simulink model "nucleo_g431re_ihm07m1"  (R2024a)
settings: Solver=FixedStepDiscrete  StartTime=0.0  StopTime=10  FixedStep=Ts  RelTol=1e-3  EnableMultiTasking=on
model workspace (MAT data in the model file):
  encoderResolution = 2000
  hallOffset = '0.5'
  indexOffset = 850
  polePairs = '4'
values from neighbouring files (symbols this model uses):
  motorParam =     [matlab.mat]
  PWM_Counter_Period = round(CPU_frequency/PWM_frequency/2)    [mcb_stm32_param_est_InitFunc.m]
  Ts = 1/PWM_frequency    (= 5e-05)    [mcb_stm32_param_est_InitFunc.m]    (also in stm32_pmsm_foc_data.m)
undefined symbols (not defined in the file or in its folder): DiscIntNeverNeededParam, inverter, NumBits1, NumBits2, Slope1, Slope2
libraries: mcbcontrolslib x24, simulink x15, stm32f4xxblockslib x4, stm32g4xxblockslib x3, slpidlib x2, stm32blockslib x2, svdutilitieslib x1
(part 2 of 3)

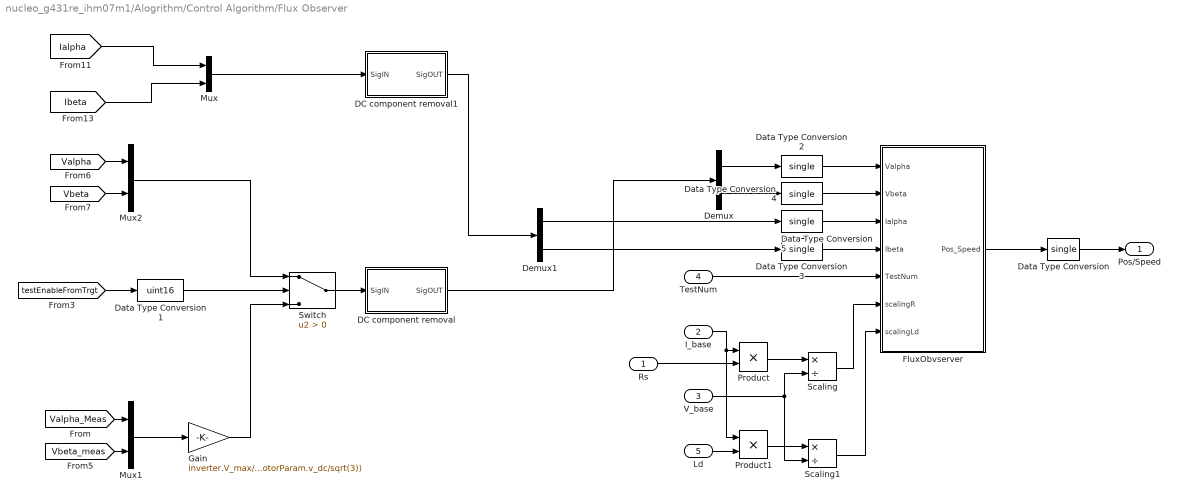
== system nucleo_g431re_ihm07m1/Alogrithm/Control Algorithm/Flux Observer ==
  Rs : Inport
  I_base : Inport  Port=2
  V_base : Inport  Port=3
  TestNum : Inport  Port=4
  Ld : Inport  Port=5
  DC component removal : Subsystem
  DC component removal1 : Subsystem
  Data Type Conversion{,2..5} (5 alike) : DataTypeConversion  OutDataTypeStr=single  RndMeth=Simplest  SaturateOnIntegerOverflow=off
  Data Type Conversion1 : DataTypeConversion  OutDataTypeStr=uint16  RndMeth=Simplest  SaturateOnIntegerOverflow=off
  Demux : Demux  Outputs=2
  Demux1 : Demux  Outputs=2
  FluxObvserver : Subsystem
  Gain : Gain  Gain=inverter.V_max/(motorParam.v_dc/sqrt(3))  RndMeth=Simplest  OutDataTypeStr=Inherit: Same as input
  Mux : Mux  Inputs=2
  Mux1 : Mux  Inputs=2
  Mux2 : Mux  Inputs=2
  Product : Product
  Product1 : Product
  Scaling : Product  Inputs=*/
  Scaling1 : Product  Inputs=*/
  Switch : Switch  Criteria=u2 > Threshold  SaturateOnIntegerOverflow=off  InputSameDT=off
  Pos/Speed : Outport  VectorParamsAs1DForOutWhenUnconnected=off
  wires:
  Data Type Conversion/1 -> Pos/Speed/1
  I_base/1 -> Product1/1, Product/1
  Rs/1 -> Product/2
  Product/1 -> Scaling/1
  [Ibeta] -> Mux/2
  [Ialpha] -> Mux/1
  Demux/2 -> Data Type Conversion4/1
  Demux/1 -> Data Type Conversion2/1
  FluxObvserver/1(Pos_Speed) -> Data Type Conversion/1
  Data Type Conversion2/1 -> FluxObvserver/1(Valpha)
  Data Type Conversion4/1 -> FluxObvserver/2(Vbeta)
  TestNum/1 -> FluxObvserver/5(TestNum)
  Scaling/1 -> FluxObvserver/6(scalingR)
  [Vbeta_meas] -> Mux1/2
  Mux1/1 -> Gain/1
  [Valpha_Meas] -> Mux1/1
  Gain/1 -> Switch/3
  V_base/1 -> Scaling/2, Scaling1/2
  Product1/1 -> Scaling1/1
  Ld/1 -> Product1/2
  Scaling1/1 -> FluxObvserver/7(scalingLd)
  Data Type Conversion1/1 -> Switch/2
  [Valpha] -> Mux2/1
  [Vbeta] -> Mux2/2
  Mux2/1 -> Switch/1
  [testEnableFromTrgt] -> Data Type Conversion1/1
  Data Type Conversion5/1 -> FluxObvserver/3(Ialpha)
  Data Type Conversion3/1 -> FluxObvserver/4(Ibeta)
  Switch/1 -> DC component removal/1(SigIN)
  DC component removal/1(SigOUT) -> Demux/1
  DC component removal1/1(SigOUT) -> Demux1/1
  Demux1/2 -> Data Type Conversion3/1
  Mux/1 -> DC component removal1/1(SigIN)
  Demux1/1 -> Data Type Conversion5/1

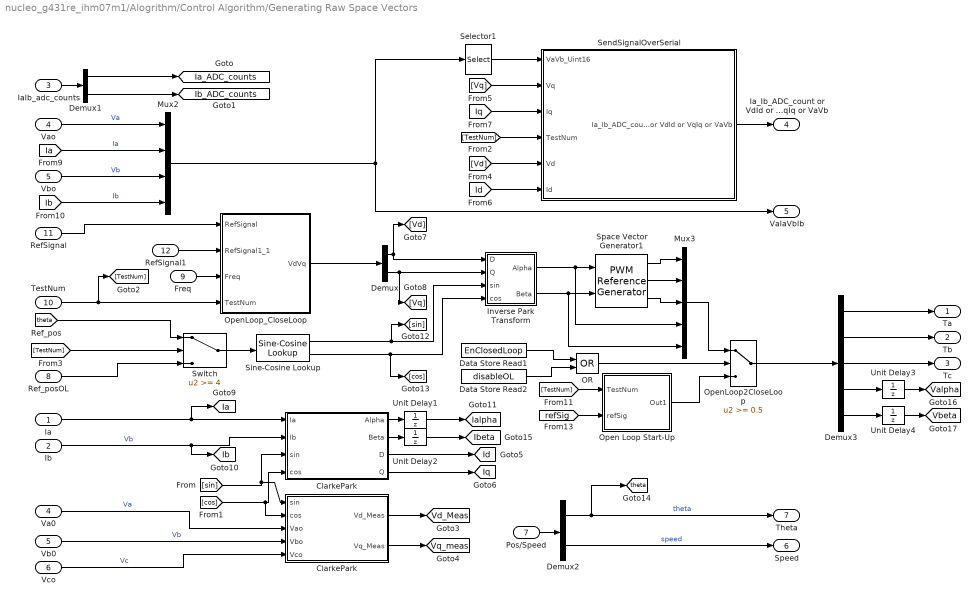
== system nucleo_g431re_ihm07m1/Alogrithm/Control Algorithm/Generating Raw Space Vectors ==
  Ia : Inport
  Ib : Inport  Port=2
  IaIb_adc_counts : Inport  Port=3
  Vao : Inport  Port=4
  Vbo : Inport  Port=5
  Vco : Inport  Port=6
  Pos/Speed : Inport  Port=7
  Ref_posOL : Inport  Port=8
  Freq : Inport  Port=9
  TestNum : Inport  Port=10
  RefSignal : Inport  Port=11
  RefSignal1 : Inport  Port=12
  ClarkePark : Subsystem
  "ClarkePark " : Subsystem
  Data Store Read1 : DataStoreRead  DataStoreName=EnClosedLoop  IndexOptions=Index vector (dialog)  Indices=1  OutputSizes=1
  Data Store Read2 : DataStoreRead  DataStoreName=disableOL  IndexOptions=Index vector (dialog)  Indices=1  OutputSizes=1
  Demux : Demux  Outputs=2
  Demux1 : Demux  Outputs=2
  Demux2 : Demux  Outputs=2
  Demux3 : Demux  Outputs=5
  Inverse Park Transform : Subsystem
  Mux2 : Mux
  Mux3 : Mux  Inputs=5
  OR : Logic  Operator=OR  IconShape=distinctive  AllPortsSameDT=off  OutDataTypeStr=boolean
  Open Loop Start-Up : Subsystem
  OpenLoop2CloseLoop : Switch  Threshold=0.5  OutDataTypeStr=Inherit: Inherit via back propagation  RndMeth=Simplest  SaturateOnIntegerOverflow=off  InputSameDT=off
  OpenLoop_CloseLoop : Subsystem
  Selector1 : Selector  InputPortWidth=4  IndexOptions=Index vector (dialog)  Indices=[1 3]  OutputSizes=1
  SendSignalOverSerial : Subsystem
  Sine-Cosine Lookup : mcbcontrolslib/Sine-Cosine Lookup  AngleInput=Per-unit  N_points=1024  DatatypeInput=Inherit from input  Datatype=single
  Space Vector Generator1 : mcbcontrolslib/PWM Reference Generator  inSignal=Valphabeta  modType=SVM: space vector modulation
  Switch : Switch  Threshold=4  SaturateOnIntegerOverflow=off  InputSameDT=off
  Unit Delay{1..4} (4 alike) : UnitDelay  SampleTime=-1  HasFrameUpgradeWarning=on
  Va0 : InportShadow  Port=4
  Vb0 : InportShadow  Port=5
  Ta : Outport  VectorParamsAs1DForOutWhenUnconnected=off
  Tb : Outport  Port=2  VectorParamsAs1DForOutWhenUnconnected=off
  Tc : Outport  Port=3  VectorParamsAs1DForOutWhenUnconnected=off
  Ia_Ib_ADC_count or VdId or VqIq or VaVb : Outport  Port=4  VectorParamsAs1DForOutWhenUnconnected=off
  VaIaVbIb : Outport  Port=5  VectorParamsAs1DForOutWhenUnconnected=off
  Speed : Outport  Port=6  VectorParamsAs1DForOutWhenUnconnected=off
  Theta : Outport  Port=7  VectorParamsAs1DForOutWhenUnconnected=off
  tag scope: Ia=global, Ia_ADC_counts=global, Ialpha=global, Ib=global, Ib_ADC_counts=global, Ibeta=global, Id=global, Iq=global, Valpha=global, Vbeta=global, Vd_Meas=global, Vq_meas=global, theta=global
  wires:
  Demux/2 -> Inverse Park Transform/2(Q), [Vq]
  Demux/1 -> Inverse Park Transform/1(D), [Vd]
  Freq/1 -> OpenLoop_CloseLoop/3(Freq)
  TestNum/1 -> [TestNum], OpenLoop_CloseLoop/4(TestNum)
  Ia/1 -> "ClarkePark "/1(Ia), [Ia]
  Ib/1 -> "ClarkePark "/2(Ib), [Ib]  "Vb"
  Demux2/1 -> [theta], Theta/1  "theta"
  RefSignal/1 -> OpenLoop_CloseLoop/1(RefSignal)
  OpenLoop_CloseLoop/1(VdVq) -> Demux/1
  Ref_posOL/1 -> Switch/3
  [TestNum] -> Switch/2
  Pos/Speed/1 -> Demux2/1
  Demux2/2 -> Speed/1  "speed"
  ClarkePark/1(Vd_Meas) -> [Vd_Meas]
  ClarkePark/2(Vq_Meas) -> [Vq_meas]
  Vb0/1 -> ClarkePark/4(Vbo)  "Vb"
  Va0/1 -> ClarkePark/3(Vao)  "Va"
  Vco/1 -> ClarkePark/5(Vco)  "Vc"
  "ClarkePark "/3(D) -> [Id]
  "ClarkePark "/4(Q) -> [Iq]
  [Iq] -> SendSignalOverSerial/3(Iq)
  [TestNum] -> SendSignalOverSerial/4(TestNum)
  [Id] -> SendSignalOverSerial/6(Id)
  SendSignalOverSerial/1(Ia_Ib_ADC_count or VdId or VqIq or VaVb) -> Ia_Ib_ADC_count or VdId or VqIq or VaVb/1
  Vao/1 -> Mux2/1  "Va"
  [Ia] -> Mux2/2  "Ia"
  Vbo/1 -> Mux2/3  "Vb"
  [Ib] -> Mux2/4  "Ib"
  Mux2/1 -> VaIaVbIb/1, Selector1/1
  Demux1/2 -> [Ib_ADC_counts]
  IaIb_adc_counts/1 -> Demux1/1
  Demux1/1 -> [Ia_ADC_counts]
  Selector1/1 -> SendSignalOverSerial/1(VaVb_Uint16)
  Switch/1 -> Sine-Cosine Lookup/1
  Sine-Cosine Lookup/1 -> Inverse Park Transform/3(sin), [sin]
  Sine-Cosine Lookup/2 -> Inverse Park Transform/4(cos), [cos]
  [theta] -> Switch/1
  [sin] -> ClarkePark/1(sin), "ClarkePark "/3(sin)
  [cos] -> ClarkePark/2(cos), "ClarkePark "/4(cos)
  [Vq] -> SendSignalOverSerial/2(Vq)
  [Vd] -> SendSignalOverSerial/5(Vd)
  Open Loop Start-Up/1(Out1) -> OpenLoop2CloseLoop/3
  [refSig] -> Open Loop Start-Up/2(refSig)
  Space Vector Generator1/1 -> Mux3/1
  Mux3/1 -> OpenLoop2CloseLoop/1
  Space Vector Generator1/2 -> Mux3/2
  Space Vector Generator1/3 -> Mux3/3
  [TestNum] -> Open Loop Start-Up/1(TestNum)
  Inverse Park Transform/2(Beta) -> Space Vector Generator1/2, Mux3/5
  Inverse Park Transform/1(Alpha) -> Space Vector Generator1/1, Mux3/4
  OpenLoop2CloseLoop/1 -> Demux3/1
  Demux3/1 -> Ta/1
  Demux3/2 -> Tb/1
  Demux3/3 -> Tc/1
  Unit Delay4/1 -> [Vbeta]
  Unit Delay3/1 -> [Valpha]
  Demux3/4 -> Unit Delay3/1
  Demux3/5 -> Unit Delay4/1
  Data Store Read1/1 -> OR/1
  Data Store Read2/1 -> OR/2
  OR/1 -> OpenLoop2CloseLoop/2
  "ClarkePark "/1(Alpha) -> Unit Delay1/1
  "ClarkePark "/2(Beta) -> Unit Delay2/1
  Unit Delay1/1 -> [Ialpha]
  Unit Delay2/1 -> [Ibeta]
  RefSignal1/1 -> OpenLoop_CloseLoop/2(RefSignal1_1)

== system nucleo_g431re_ihm07m1/Alogrithm/Control Algorithm/Voltage Scaling ==
  Vabc : Inport
  Data Type Conversion4 : DataTypeConversion  OutDataTypeStr=single  RndMeth=Simplest  SaturateOnIntegerOverflow=off
  Demux : Demux
  Gain : Gain  Commented=through  Gain=1/0.0522  OutDataTypeStr=Inherit: Same as input  ParamDataTypeStr=Inherit: Same as input
  count_to_PU : Gain  Gain=1/4096  OutDataTypeStr=single  RndMeth=Simplest
  Vao : Outport  VectorParamsAs1DForOutWhenUnconnected=off
  Vbo : Outport  Port=2  VectorParamsAs1DForOutWhenUnconnected=off
  Vco : Outport  Port=3  VectorParamsAs1DForOutWhenUnconnected=off
  Vdc : Outport  Port=4  VectorParamsAs1DForOutWhenUnconnected=off
  wires:
  Demux/3 -> Vco/1
  Demux/1 -> Vao/1
  Demux/2 -> Vbo/1
  Demux/4 -> Gain/1
  count_to_PU/1 -> Demux/1
  Data Type Conversion4/1 -> count_to_PU/1
  Vabc/1 -> Data Type Conversion4/1
  Gain/1 -> Vdc/1

== system nucleo_g431re_ihm07m1/Alogrithm/PWM_HW/PWM scaling ==
  Ta/Tb/Tc : Inport
  Add : Sum
  Constant : Constant  OutDataTypeStr=single
  Data Store Read : DataStoreRead  DataStoreName=testEnableFromHost  IndexOptions=Index vector (dialog)  Indices=1  OutputSizes=1
  Data Type Conversion : DataTypeConversion  OutDataTypeStr=uint16  SaturateOnIntegerOverflow=off  RndMeth=Floor
  Mux2 : Mux  Inputs=3
  PWM_Counter_Period : Gain  Gain=PWM_Counter_Period/2  ParamDataTypeStr=single  OutDataTypeStr=single  RndMeth=Simplest
  Switch1 : Switch  Threshold=0.5  RndMeth=Simplest  SaturateOnIntegerOverflow=off  InputSameDT=off
  stop : Constant  Value=0  OutDataTypeStr=single
  PWM A/B/C : Outport  VectorParamsAs1DForOutWhenUnconnected=off
  wires:
  Constant/1 -> Add/1
  Ta/Tb/Tc/1 -> Add/2
  PWM_Counter_Period/1 -> Data Type Conversion/1
  Add/1 -> PWM_Counter_Period/1
  Data Type Conversion/1 -> Switch1/1
  Switch1/1 -> PWM A/B/C/1
  Data Store Read/1 -> Switch1/2  "PWM_Enable"
  stop/1 -> Mux2/3, Mux2/2, Mux2/1
  Mux2/1 -> Switch1/3

== system nucleo_g431re_ihm07m1/Alogrithm/ParameterEstimationTests/Algorithm Parameters ==
  Data Store Read : DataStoreRead  DataStoreName=Vd_ref_OL  IndexOptions=Index vector (dialog)  Indices=1  OutputSizes=1
  Data Store Read1 : DataStoreRead  DataStoreName=freq_low  IndexOptions=Index vector (dialog)  Indices=1  OutputSizes=1
  Data Store Read2 : DataStoreRead  DataStoreName=freq_high  IndexOptions=Index vector (dialog)  Indices=1  OutputSizes=1
  Data Store Read3 : DataStoreRead  DataStoreName=freq_step  IndexOptions=Index vector (dialog)  Indices=1  OutputSizes=1
  Data Store Read4 : DataStoreRead  DataStoreName=Vd_dc  IndexOptions=Index vector (dialog)  Indices=1  OutputSizes=1
  Data Store Read5 : DataStoreRead  DataStoreName=Vdq_amp  IndexOptions=Index vector (dialog)  Indices=1  OutputSizes=1
  Data Store Read6 : DataStoreRead  DataStoreName=Iq_ref_CL  IndexOptions=Index vector (dialog)  Indices=1  OutputSizes=1
  Data Store Read7 : DataStoreRead  DataStoreName=under_voltage_limit  IndexOptions=Index vector (dialog)  Indices=1  OutputSizes=1
  Data Store Read8 : DataStoreRead  DataStoreName=over_current_limit  IndexOptions=Index vector (dialog)  Indices=1  OutputSizes=1
  Data Store Read9 : DataStoreRead  DataStoreName=inertia_end_speed  IndexOptions=Index vector (dialog)  Indices=1  OutputSizes=1
  Mux : Mux  Inputs=10
  AlgoParams : Outport
  wires:
  Mux/1 -> AlgoParams/1
  Data Store Read7/1 -> Mux/8
  Data Store Read8/1 -> Mux/9
  Data Store Read2/1 -> Mux/3
  Data Store Read5/1 -> Mux/6
  Data Store Read/1 -> Mux/1
  Data Store Read1/1 -> Mux/2
  Data Store Read3/1 -> Mux/4
  Data Store Read4/1 -> Mux/5
  Data Store Read6/1 -> Mux/7
  Data Store Read9/1 -> Mux/10

== system nucleo_g431re_ihm07m1/Alogrithm/ParameterEstimationTests/Triggered Subsystem ==
  Trigger : TriggerPort  VariantControl=Variant
  Constant : Constant  Value=0  OutDataTypeStr=single  SampleTime=-1
  Data Store Write1 : DataStoreWrite  DataStoreName=testEnableFromHost  IndexOptions=Index vector (dialog)  Indices=1  OutputSizes=1
  wires:
  Constant/1 -> Data Store Write1/1

== system nucleo_g431re_ihm07m1/Alogrithm/ParameterEstimationTests/counter ==
  Ts : Inport
  testEnableFromHost : Inport  Port=2
  Sum : Sum  Inputs=|++  RndMeth=Simplest  OutDataTypeStr=Inherit: Same as first input
  Switch : Switch  Criteria=u2 > Threshold  SaturateOnIntegerOverflow=off  InputSameDT=off
  Unit Delay8 : UnitDelay  SampleTime=-1  HasFrameUpgradeWarning=on
  curTime : Outport
  wires:
  Ts/1 -> Sum/1
  Sum/1 -> curTime/1, Unit Delay8/1  "curTime"
  Unit Delay8/1 -> Switch/1
  Switch/1 -> Sum/2
  testEnableFromHost/1 -> Switch/2, Switch/3

== system nucleo_g431re_ihm07m1/Alogrithm/Reference signal conditioning/Torque_control_with_speed_limit ==
  MaxSpeed : Inport
  IqRef : Inport  Port=2
  ActSpeed : Inport  Port=3
  En : Inport  Port=4
  Enable : EnablePort
  Data Store Read : DataStoreRead  DataStoreName=I_rated  IndexOptions=Index vector (dialog)  Indices=1  OutputSizes=1
  Data Store Read1 : DataStoreRead  DataStoreName=currentPU_RWV  IndexOptions=Index vector (dialog)  Indices=1  OutputSizes=1
  Data Type Conversion : DataTypeConversion  OutDataTypeStr=single  SaturateOnIntegerOverflow=off  RndMeth=Floor
  Data Type Conversion1 : DataTypeConversion  OutDataTypeStr=single  SaturateOnIntegerOverflow=off  RndMeth=Floor
  Derating Function : mcbcontrolslib/Derating Function  x=0.9
  Divide : Product  Inputs=*/  RndMeth=Simplest  OutDataTypeStr=Inherit: Same as first input
  Product : Product  Inputs=3
  Product1 : Product  OutDataTypeStr=single  RndMeth=Simplest
  Iq_ref : Outport
  wires:
  Product1/1 -> Divide/1
  Derating Function/1 -> Product/2
  Data Type Conversion/1 -> Derating Function/2
  Divide/1 -> Product/1
  Product/1 -> Iq_ref/1
  Data Store Read1/1 -> Divide/2
  Data Type Conversion1/1 -> Derating Function/1
  ActSpeed/1 -> Data Type Conversion/1
  MaxSpeed/1 -> Data Type Conversion1/1
  En/1 -> Product/3
  Data Store Read/1 -> Product1/2
  IqRef/1 -> Product1/1

== system nucleo_g431re_ihm07m1/Alogrithm/SaveEstParam_Serial Send/ChangeDetect ==
  Sig : Inport
  Equal : RelationalOperator  Operator=~=  OutDataTypeStr=boolean  RndMeth=Simplest  InputSameDT=off
  Unit Delay : UnitDelay  SampleTime=-1  HasFrameUpgradeWarning=on
  ChangeDet : Outport
  wires:
  Equal/1 -> ChangeDet/1
  Sig/1 -> Equal/2, Unit Delay/1
  Unit Delay/1 -> Equal/1

== system nucleo_g431re_ihm07m1/Alogrithm/SaveEstParam_Serial Send/SaveToMemory ==
  estimatedParameter : Inport
  estParIdx : Inport  Port=2
  Trigger : TriggerPort  TriggerType=either  VariantControl=Variant  PortDimensions=1
  B : Subsystem  TreatAsAtomicUnit=on
  Bemf : Subsystem  TreatAsAtomicUnit=on
  ErrorCase : Subsystem  TreatAsAtomicUnit=on
  Ia_cal_val : Subsystem  TreatAsAtomicUnit=on
  Ib_cal_val : Subsystem  TreatAsAtomicUnit=on
  J : Subsystem  TreatAsAtomicUnit=on
  Ld : Subsystem  TreatAsAtomicUnit=on
  Lq : Subsystem  TreatAsAtomicUnit=on
  PhaseDiffValidity : Subsystem  TreatAsAtomicUnit=on
  Rs : Subsystem  TreatAsAtomicUnit=on
  Switch Case : SwitchCase  CaseConditions={0 1 2 3 4 5 6 7 8 9}  ShowDefaultCase=off
  Idx : Outport  InitialOutput=[20]
  EstPar : Outport  Port=2  InitialOutput=[0]
  wires:
  Switch Case/9 -> ErrorCase/Action
  Switch Case/7 -> J/Action
  Switch Case/8 -> B/Action
  Switch Case/6 -> Bemf/Action
  estimatedParameter/1 -> PhaseDiffValidity/1(1), ErrorCase/1(In1), B/1(In1), J/1(In1), Bemf/1(In1), Lq/1(In1), Ld/1(In1), Rs/1(In1), Ib_cal_val/1(In1), Ia_cal_val/1(In1), EstPar/1
  estParIdx/1 -> Idx/1, Switch Case/1
  Switch Case/4 -> Ld/Action
  Switch Case/3 -> Rs/Action
  Switch Case/2 -> Ib_cal_val/Action
  Switch Case/1 -> Ia_cal_val/Action
  Switch Case/5 -> Lq/Action
  Switch Case/10 -> PhaseDiffValidity/Action

== system nucleo_g431re_ihm07m1/Alogrithm/SaveEstParam_Serial Send/Serial Send ==
  Idx : Inport
  estimatedParameter : Inport  Port=2
  SelSig : Inport  Port=3
  AlternateData : Subsystem
  Byte Pack : svdutilitieslib/Byte Pack  maskPackedDataType=uint32  datatypes={'single'}  byteAlign=4  blockPlatform=tic2000
  Data Type Conversion5 : DataTypeConversion  OutDataTypeStr=single  RndMeth=Simplest  SaturateOnIntegerOverflow=off
  Mux1 : Mux  Inputs=2
  Serial Send : Subsystem
  wires:
  Mux1/1 -> Byte Pack/1
  Idx/1 -> AlternateData/2(EstParaIdx)
  SelSig/1 -> Data Type Conversion5/1
  Data Type Conversion5/1 -> Mux1/2
  estimatedParameter/1 -> AlternateData/1(EstPara)
  AlternateData/1(Out1) -> Mux1/1
  Byte Pack/1 -> Serial Send/1(In1)

== system nucleo_g431re_ihm07m1/SerialReceive/Rx_single/Enabled Subsystem ==
  In1 : Inport
  Enable : EnablePort
  Out1 : Outport
  wires:
  In1/1 -> Out1/1

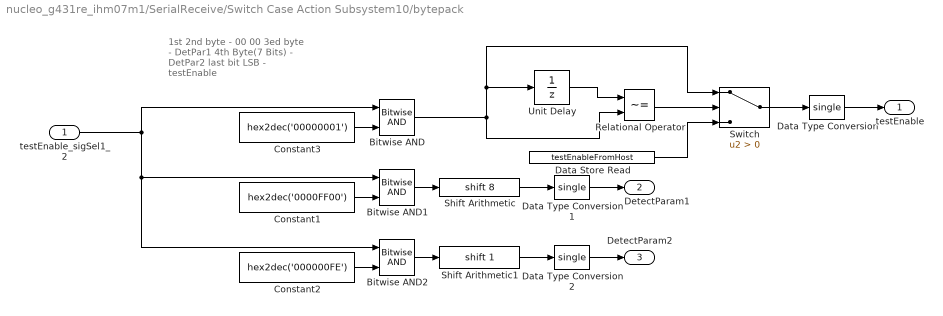
== system nucleo_g431re_ihm07m1/SerialReceive/Switch Case Action Subsystem10/bytepack ==
  note: 1st 2nd byte - 00 00
      | 3ed byte - DetPar1
      | 4th Byte(7 Bits) - DetPar2
      | last bit LSB - testEnable
  testEnable_sigSel1_2 : Inport
  Bitwise AND : simulink/Logic and Bit Operations/Bitwise Operator  logicop=AND  UseBitMask=off  NumInputPorts=2  BitMask=bin2dec('00001111')  BitMaskRealWorld=Stored Integer
  Bitwise AND1 : simulink/Logic and Bit Operations/Bitwise Operator  logicop=AND  UseBitMask=off  NumInputPorts=2  BitMask=bin2dec('00001111')  BitMaskRealWorld=Stored Integer
  Bitwise AND2 : simulink/Logic and Bit Operations/Bitwise Operator  logicop=AND  UseBitMask=off  NumInputPorts=2  BitMask=bin2dec('00001111')  BitMaskRealWorld=Stored Integer
  Constant1 : Constant  Value=hex2dec('0000FF00')  OutDataTypeStr=uint32  SampleTime=-1
  Constant2 : Constant  Value=hex2dec('000000FE')  OutDataTypeStr=uint32  SampleTime=-1
  Constant3 : Constant  Value=hex2dec('00000001')  OutDataTypeStr=uint32  SampleTime=-1
  Data Store Read : DataStoreRead  DataStoreName=testEnableFromHost  IndexOptions=Index vector (dialog)  Indices=1  OutputSizes=1
  Data Type Conversion : DataTypeConversion  OutDataTypeStr=single  RndMeth=Simplest  SaturateOnIntegerOverflow=off
  Data Type Conversion1 : DataTypeConversion  OutDataTypeStr=single  RndMeth=Simplest  SaturateOnIntegerOverflow=off
  Data Type Conversion2 : DataTypeConversion  OutDataTypeStr=single  RndMeth=Simplest  SaturateOnIntegerOverflow=off
  Relational Operator : RelationalOperator  Operator=~=  OutDataTypeStr=boolean  RndMeth=Simplest  InputSameDT=off
  Shift Arithmetic : ArithShift  BitShiftNumber=8
  Shift Arithmetic1 : ArithShift  BitShiftNumber=1
  Switch : Switch  Criteria=u2 > Threshold  SaturateOnIntegerOverflow=off  InputSameDT=off
  Unit Delay : UnitDelay  SampleTime=-1  HasFrameUpgradeWarning=on
  testEnable : Outport
  DetectParam1 : Outport  Port=2
  DetectParam2 : Outport  Port=3
  wires:
  Bitwise AND2/1 -> Shift Arithmetic1/1
  Bitwise AND1/1 -> Shift Arithmetic/1
  Bitwise AND/1 -> Switch/1, Unit Delay/1, Relational Operator/2
  Constant3/1 -> Bitwise AND/2
  Constant1/1 -> Bitwise AND1/2
  Constant2/1 -> Bitwise AND2/2
  Data Type Conversion/1 -> testEnable/1
  Data Type Conversion1/1 -> DetectParam1/1
  Data Type Conversion2/1 -> DetectParam2/1
  testEnable_sigSel1_2/1 -> Bitwise AND2/1, Bitwise AND1/1, Bitwise AND/1
  Shift Arithmetic1/1 -> Data Type Conversion2/1
  Shift Arithmetic/1 -> Data Type Conversion1/1
  Unit Delay/1 -> Relational Operator/1
  Relational Operator/1 -> Switch/2
  Switch/1 -> Data Type Conversion/1
  Data Store Read/1 -> Switch/3

== system nucleo_g431re_ihm07m1/Alogrithm/Control Algorithm/Flux Observer/DC component removal ==
  SigIN : Inport
  IIR Filter : mcbcontrolslib/IIR Filter  VariantControl=Low Pass Filter  VariantSelect=Low-pass  FilterConstantInputType=Specify via dialog  Filter_constant=0.005*(Ts/50e-6)  advancedSettings=off  Ts=50e-6  cutOff_freq=32.1525
  Sum6 : Sum  Inputs=|+-  RndMeth=Simplest  OutDataTypeStr=Inherit: Same as first input
  SigOUT : Outport
  wires:
  IIR Filter/1 -> Sum6/2
  SigIN/1 -> IIR Filter/1, Sum6/1
  Sum6/1 -> SigOUT/1

== system nucleo_g431re_ihm07m1/Alogrithm/Control Algorithm/Flux Observer/DC component removal1 ==
  SigIN : Inport
  IIR Filter : mcbcontrolslib/IIR Filter  VariantControl=Low Pass Filter  VariantSelect=Low-pass  FilterConstantInputType=Specify via dialog  Filter_constant=0.005*(Ts/50e-6)  advancedSettings=off  Ts=50e-6  cutOff_freq=32.1525
  Sum6 : Sum  Inputs=|+-  RndMeth=Simplest  OutDataTypeStr=Inherit: Same as first input
  SigOUT : Outport
  wires:
  IIR Filter/1 -> Sum6/2
  SigIN/1 -> IIR Filter/1, Sum6/1
  Sum6/1 -> SigOUT/1

== system nucleo_g431re_ihm07m1/Alogrithm/Control Algorithm/Flux Observer/FluxObvserver ==
  Valpha : Inport
  Vbeta : Inport  Port=2
  Ialpha : Inport  Port=3
  Ibeta : Inport  Port=4
  TestNum : Inport  Port=5
  scalingR : Inport  Port=6
  scalingLd : Inport  Port=7
  Compare To Constant : simulink/Logic and Bit Operations/Compare To Constant  relop=>=  const=4  OutDataTypeStr=boolean
  FluxObserverSubsystem : Subsystem
  Gain1 : Gain  Commented=through  Gain=2  RndMeth=Simplest  OutDataTypeStr=Inherit: Same as input
  Gain2 : Gain  Commented=through  Gain=2  RndMeth=Simplest  OutDataTypeStr=Inherit: Same as input
  Mux2 : Mux  Inputs=2
  NOT : Logic  Operator=NOT  IconShape=distinctive  AllPortsSameDT=off  OutDataTypeStr=boolean
  SpeedMeasurementSubsystem : Subsystem
  Pos_Speed : Outport
  wires:
  NOT/1 -> FluxObserverSubsystem/5(Reset)
  Ibeta/1 -> Gain2/1
  scalingR/1 -> FluxObserverSubsystem/6(scaling)
  Valpha/1 -> SpeedMeasurementSubsystem/1(V_alpha), FluxObserverSubsystem/1(Valpha)
  Ialpha/1 -> Gain1/1
  Vbeta/1 -> SpeedMeasurementSubsystem/2(V_beta), FluxObserverSubsystem/2(Vbeta)
  Mux2/1 -> Pos_Speed/1
  scalingLd/1 -> FluxObserverSubsystem/7(scalingLd)
  Compare To Constant/1 -> NOT/1
  TestNum/1 -> Compare To Constant/1
  SpeedMeasurementSubsystem/1(Speed) -> Mux2/2
  Gain1/1 -> FluxObserverSubsystem/3(Ialpha)
  Gain2/1 -> FluxObserverSubsystem/4(Ibeta)
  FluxObserverSubsystem/1(Position) -> Mux2/1

== system nucleo_g431re_ihm07m1/Alogrithm/Control Algorithm/Generating Raw Space Vectors/ClarkePark ==
  sin : Inport
  cos : Inport  Port=2
  Vao : Inport  Port=3
  Vbo : Inport  Port=4
  Vco : Inport  Port=5
  Clarke Transform : mcbcontrolslib/Clarke Transform  VariantControl=Variant2  PhaseInput=Two inputs  EnPowerInv=off
  Park Transform : mcbcontrolslib/Park Transform  PhaseInput=Two inputs  AxisAlignment=D-axis  ThetaInput=Sine and Cosine electrical position  AngleInput=Per-unit  N_points=1024
  Pole_Voltage to Phase_Voltage : Subsystem
  Vd_Meas : Outport  VectorParamsAs1DForOutWhenUnconnected=off
  Vq_Meas : Outport  Port=2  VectorParamsAs1DForOutWhenUnconnected=off
  tag scope: Valpha_Meas=global, Vbeta_meas=global
  wires:
  Vco/1 -> Pole_Voltage to Phase_Voltage/3(Vco)
  Clarke Transform/2 -> Park Transform/2, [Vbeta_meas]
  Pole_Voltage to Phase_Voltage/1(Va) -> Clarke Transform/1
  Park Transform/2 -> Vq_Meas/1  "Vq"
  Clarke Transform/1 -> [Valpha_Meas], Park Transform/1
  Pole_Voltage to Phase_Voltage/2(Vb) -> Clarke Transform/2
  Park Transform/1 -> Vd_Meas/1  "Vd"
  Vbo/1 -> Pole_Voltage to Phase_Voltage/2(Vbo)
  Vao/1 -> Pole_Voltage to Phase_Voltage/1(Vao)
  sin/1 -> Park Transform/3
  cos/1 -> Park Transform/4

== system nucleo_g431re_ihm07m1/Alogrithm/Control Algorithm/Generating Raw Space Vectors/ClarkePark  ==
  Ia : Inport
  Ib : Inport  Port=2
  sin : Inport  Port=3
  cos : Inport  Port=4
  Clarke Transform : mcbcontrolslib/Clarke Transform  VariantControl=Variant2  PhaseInput=Two inputs  EnPowerInv=off
  Park Transform : mcbcontrolslib/Park Transform  PhaseInput=Two inputs  AxisAlignment=D-axis  ThetaInput=Sine and Cosine electrical position  AngleInput=Per-unit  N_points=1024
  Alpha : Outport  VectorParamsAs1DForOutWhenUnconnected=off
  Beta : Outport  Port=2  VectorParamsAs1DForOutWhenUnconnected=off
  D : Outport  Port=3  VectorParamsAs1DForOutWhenUnconnected=off
  Q : Outport  Port=4  VectorParamsAs1DForOutWhenUnconnected=off
  wires:
  Clarke Transform/1 -> Park Transform/1, Alpha/1
  Park Transform/1 -> D/1  "Va"
  Clarke Transform/2 -> Park Transform/2, Beta/1
  Park Transform/2 -> Q/1
  Ib/1 -> Clarke Transform/2
  Ia/1 -> Clarke Transform/1
  sin/1 -> Park Transform/3
  cos/1 -> Park Transform/4

== system nucleo_g431re_ihm07m1/Alogrithm/Control Algorithm/Generating Raw Space Vectors/Inverse Park Transform ==
  D : Inport
  Q : Inport  Port=2
  sin : Inport  Port=3
  cos : Inport  Port=4
  Inverse Park Transform : mcbcontrolslib/Inverse Park Transform  PhaseInput=Two inputs  AxisAlignment=D-axis  ThetaInput=Sine and Cosine electrical position  AngleInput=Per-unit  N_points=1024
  Alpha : Outport  VectorParamsAs1DForOutWhenUnconnected=off
  Beta : Outport  Port=2  VectorParamsAs1DForOutWhenUnconnected=off
  wires:
  Inverse Park Transform/2 -> Beta/1
  sin/1 -> Inverse Park Transform/3
  Q/1 -> Inverse Park Transform/2
  cos/1 -> Inverse Park Transform/4
  Inverse Park Transform/1 -> Alpha/1
  D/1 -> Inverse Park Transform/1

== system nucleo_g431re_ihm07m1/Alogrithm/Control Algorithm/Generating Raw Space Vectors/Open Loop Start-Up ==
  TestNum : Inport
  refSig : Inport  Port=2
  Compare To Constant1 : simulink/Logic and Bit Operations/Compare To Constant  relop=>=  const=4  OutDataTypeStr=boolean
  Data Store Write : DataStoreWrite  DataStoreName=disableOL  IndexOptions=Index vector (dialog)  Indices=1  OutputSizes=1
  Mux1 : Mux  Inputs=2
  NOT : Logic  Operator=NOT  IconShape=distinctive  AllPortsSameDT=off  OutDataTypeStr=boolean
  Open Loop Start-Up : Subsystem
  Unit Delay : UnitDelay  SampleTime=-1  HasFrameUpgradeWarning=on
  Out1 : Outport
  wires:
  Unit Delay/1 -> Open Loop Start-Up/1(Enable)
  Compare To Constant1/1 -> NOT/1, Open Loop Start-Up/Enable, Unit Delay/1
  Open Loop Start-Up/2(Vfb_openloop) -> Mux1/2
  Open Loop Start-Up/1(Duty Cycles) -> Mux1/1
  refSig/1 -> Open Loop Start-Up/2(refSig)
  TestNum/1 -> Compare To Constant1/1
  NOT/1 -> Data Store Write/1
  Mux1/1 -> Out1/1

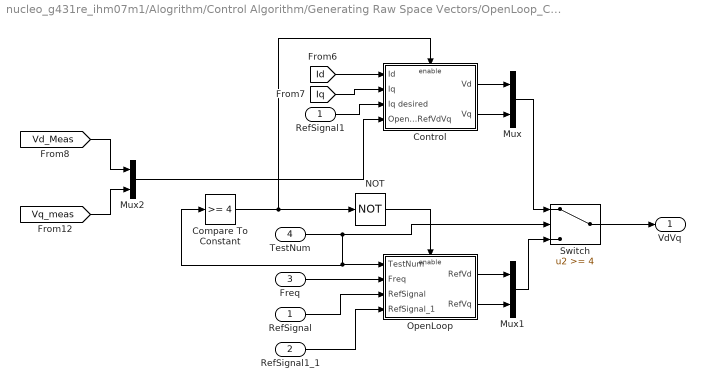
== system nucleo_g431re_ihm07m1/Alogrithm/Control Algorithm/Generating Raw Space Vectors/OpenLoop_CloseLoop ==
  RefSignal : Inport
  RefSignal1_1 : Inport  Port=2
  Freq : Inport  Port=3
  TestNum : Inport  Port=4
  Compare To Constant : simulink/Logic and Bit Operations/Compare To Constant  relop=>=  const=4  OutDataTypeStr=boolean
  Control : Subsystem
  Mux : Mux  Inputs=2
  Mux1 : Mux  Inputs=2
  Mux2 : Mux  Inputs=2
  NOT : Logic  Operator=NOT  IconShape=distinctive  AllPortsSameDT=off  OutDataTypeStr=boolean
  OpenLoop : Subsystem
  RefSignal1 : InportShadow
  Switch : Switch  Threshold=4  SaturateOnIntegerOverflow=off  InputSameDT=off
  VdVq : Outport  VectorParamsAs1DForOutWhenUnconnected=off
  wires:
  Freq/1 -> OpenLoop/2(Freq)
  TestNum/1 -> Compare To Constant/1, OpenLoop/1(TestNum), Switch/2
  [Iq] -> Control/2(Iq)
  [Id] -> Control/1(Id)
  Control/1(Vd) -> Mux/1
  Control/2(Vq) -> Mux/2
  OpenLoop/1(RefVd) -> Mux1/1
  OpenLoop/2(RefVq) -> Mux1/2
  Mux/1 -> Switch/1
  Mux1/1 -> Switch/3
  NOT/1 -> OpenLoop/Enable
  RefSignal1/1 -> Control/3(Iq desired)
  RefSignal/1 -> OpenLoop/3(RefSignal)
  RefSignal1_1/1 -> OpenLoop/4(RefSignal_1)
  Switch/1 -> VdVq/1
  Compare To Constant/1 -> Control/Enable, NOT/1
  Mux2/1 -> Control/4(OpenLoop_RefVdVq)
  [Vd_Meas] -> Mux2/1
  [Vq_meas] -> Mux2/2

== system nucleo_g431re_ihm07m1/Alogrithm/Control Algorithm/Generating Raw Space Vectors/SendSignalOverSerial ==
  VaVb_Uint16 : Inport
  Vq : Inport  Port=2
  Iq : Inport  Port=3
  TestNum : Inport  Port=4
  Vd : Inport  Port=5
  Id : Inport  Port=6
  Multiport Switch : MultiPortSwitch  DataPortOrder=Specify indices  Inputs=2  DataPortIndices={4,3,2,1,0}  OutDataTypeStr=single  RndMeth=Simplest  SaturateOnIntegerOverflow=off  InputSameDT=off
  Mux : Mux  Inputs=2
  Mux1 : Mux  Inputs=2
  Mux3 : Mux  Inputs=2
  Ia_Ib_ADC_count or VdId or VqIq or VaVb : Outport  OutDataTypeStr=single  VectorParamsAs1DForOutWhenUnconnected=off
  tag scope: VdId_32_Q17=global, VdIduint16=global, VqIq_32_Q17=global, VqIquint16=global
  wires:
  Mux/1 -> [VdIduint16], Multiport Switch/5, Multiport Switch/4, [VdId_32_Q17]
  Iq/1 -> Mux3/2  "Iq"
  Vq/1 -> Mux3/1  "Vq"
  Vd/1 -> Mux/1  "Vd"
  TestNum/1 -> Multiport Switch/1
  Mux3/1 -> [VqIq_32_Q17], [VqIquint16], Multiport Switch/3
  Id/1 -> Mux/2  "Id"
  Multiport Switch/1 -> Ia_Ib_ADC_count or VdId or VqIq or VaVb/1
  VaVb_Uint16/1 -> Multiport Switch/2
  Mux1/1 -> Multiport Switch/6
  [Ia_ADC_counts] -> Mux1/1
  [Ib_ADC_counts] -> Mux1/2

== system nucleo_g431re_ihm07m1/Alogrithm/SaveEstParam_Serial Send/SaveToMemory/B ==
  In1 : Inport
  Action Port : ActionPort  ActionPortLabel=case [ 7 ]:
  Data Store Write3 : DataStoreWrite  DataStoreName=B  IndexOptions=Index vector (dialog)  Indices=1  OutputSizes=1
  wires:
  In1/1 -> Data Store Write3/1

== system nucleo_g431re_ihm07m1/Alogrithm/SaveEstParam_Serial Send/SaveToMemory/Bemf ==
  In1 : Inport
  Action Port : ActionPort  ActionPortLabel=case [ 5 ]:
  Data Store Write3 : DataStoreWrite  DataStoreName=Bemf  IndexOptions=Index vector (dialog)  Indices=1  OutputSizes=1
  wires:
  In1/1 -> Data Store Write3/1

== system nucleo_g431re_ihm07m1/Alogrithm/SaveEstParam_Serial Send/SaveToMemory/ErrorCase ==
  In1 : Inport
  Action Port : ActionPort  ActionPortLabel=case [ 8 ]:
  Data Store Write3 : DataStoreWrite  DataStoreName=errorID  IndexOptions=Index vector (dialog)  Indices=1  OutputSizes=1
  wires:
  In1/1 -> Data Store Write3/1

== system nucleo_g431re_ihm07m1/Alogrithm/SaveEstParam_Serial Send/SaveToMemory/Ia_cal_val ==
  In1 : Inport
  Action Port : ActionPort  ActionPortLabel=case [ 0 ]:
  Data Store Write1 : DataStoreWrite  DataStoreName=Ia_avg_cal  IndexOptions=Index vector (dialog)  Indices=1  OutputSizes=1
  Gain : Gain  Gain=1e4  RndMeth=Simplest  OutDataTypeStr=Inherit: Same as input
  wires:
  In1/1 -> Gain/1
  Gain/1 -> Data Store Write1/1

== system nucleo_g431re_ihm07m1/Alogrithm/SaveEstParam_Serial Send/SaveToMemory/Ib_cal_val ==
  In1 : Inport
  Action Port : ActionPort  ActionPortLabel=case [ 1 ]:
  Data Store Write2 : DataStoreWrite  DataStoreName=Ib_avg_cal  IndexOptions=Index vector (dialog)  Indices=1  OutputSizes=1
  Gain : Gain  Gain=1e4  RndMeth=Simplest  OutDataTypeStr=Inherit: Same as input
  wires:
  In1/1 -> Gain/1
  Gain/1 -> Data Store Write2/1

== system nucleo_g431re_ihm07m1/Alogrithm/SaveEstParam_Serial Send/SaveToMemory/J ==
  In1 : Inport
  Action Port : ActionPort  ActionPortLabel=case [ 6 ]:
  Data Store Write3 : DataStoreWrite  DataStoreName=J  IndexOptions=Index vector (dialog)  Indices=1  OutputSizes=1
  wires:
  In1/1 -> Data Store Write3/1

== system nucleo_g431re_ihm07m1/Alogrithm/SaveEstParam_Serial Send/SaveToMemory/Ld ==
  In1 : Inport
  Action Port : ActionPort  ActionPortLabel=case [ 3 ]:
  Data Store Write4 : DataStoreWrite  DataStoreName=Ld  IndexOptions=Index vector (dialog)  Indices=1  OutputSizes=1
  wires:
  In1/1 -> Data Store Write4/1

== system nucleo_g431re_ihm07m1/Alogrithm/SaveEstParam_Serial Send/SaveToMemory/Lq ==
  In1 : Inport
  Action Port : ActionPort  ActionPortLabel=case [ 4 ]:
  Data Store Write3 : DataStoreWrite  DataStoreName=Lq  IndexOptions=Index vector (dialog)  Indices=1  OutputSizes=1
  wires:
  In1/1 -> Data Store Write3/1

== system nucleo_g431re_ihm07m1/Alogrithm/SaveEstParam_Serial Send/SaveToMemory/PhaseDiffValidity ==
  1 : Inport
  Action Port : ActionPort  ActionPortLabel=case [ 9 ]:
  Data Store Write : DataStoreWrite  DataStoreName=PhaseDiffValid  IndexOptions=Index vector (dialog)  Indices=1  OutputSizes=1
  wires:
  1/1 -> Data Store Write/1

== system nucleo_g431re_ihm07m1/Alogrithm/SaveEstParam_Serial Send/SaveToMemory/Rs ==
  In1 : Inport
  Action Port : ActionPort  ActionPortLabel=case [ 2 ]:
  Data Store Write2 : DataStoreWrite  DataStoreName=Rs  IndexOptions=Index vector (dialog)  Indices=1  OutputSizes=1
  wires:
  In1/1 -> Data Store Write2/1

== system nucleo_g431re_ihm07m1/Alogrithm/SaveEstParam_Serial Send/Serial Send/AlternateData ==
  EstPara : Inport
  EstParaIdx : Inport  Port=2
  Alternate_0_2 : Subsystem
  Data Type Conversion5 : DataTypeConversion  OutDataTypeStr=single  RndMeth=Simplest  SaturateOnIntegerOverflow=off
  Switch : Switch  Criteria=u2 ~= 0  SaturateOnIntegerOverflow=off  InputSameDT=off
  Out1 : Outport
  wires:
  EstParaIdx/1 -> Switch/3
  Data Type Conversion5/1 -> Out1/1
  Switch/1 -> Data Type Conversion5/1
  EstPara/1 -> Switch/1
  Alternate_0_2/1(Out1) -> Switch/2

== system nucleo_g431re_ihm07m1/Alogrithm/SaveEstParam_Serial Send/Serial Send/Serial Send ==
  In1 : Inport
  Counter Limited : simulink/Sources/Counter Limited  uplimit=599  tsamp=-1
  Data : Subsystem  TreatAsAtomicUnit=on
  End : Subsystem  TreatAsAtomicUnit=on
  If : If  IfExpression=u1 == 0  ElseIfExpressions=u1 == 599
  Merge : Merge  Inputs=3
  Merge1 : Merge  Inputs=3
  Start : Subsystem  TreatAsAtomicUnit=on
  While Iterator Subsystem : Subsystem  TreatAsAtomicUnit=on
  Width : Width  OutDataTypeMode=All ports same datatype  DataType=uint16
  wires:
  If/1 -> Start/Action
  If/2 -> End/Action
  If/3 -> Data/Action
  Counter Limited/1 -> If/1
  Start/1(Data_out) -> Merge/1
  End/1(Data_out) -> Merge/2
  Data/1(Data_out) -> Merge/3
  Merge/1 -> While Iterator Subsystem/1(Data)
  Merge1/1 -> While Iterator Subsystem/2(Iteration)
  Start/2(Iteration) -> Merge1/1
  End/2(Iteration) -> Merge1/2
  Data/2(Iteration) -> Merge1/3
  In1/1 -> Width/1, Start/1(Data), End/1(Data), Data/1(Data)
  Width/1 -> Data/2(Data_width), Start/2(Data_width), End/2(Data_width)

== system nucleo_g431re_ihm07m1/Alogrithm/Control Algorithm/Flux Observer/FluxObvserver/FluxObserverSubsystem ==
  note: Position Calculation
  Valpha : Inport
  Vbeta : Inport  Port=2
  Ialpha : Inport  Port=3
  Ibeta : Inport  Port=4
  Reset : Inport  Port=5
  scaling : Inport  Port=6
  scalingLd : Inport  Port=7
  PositionGain : Gain  OutDataTypeStr=single  RndMeth=Simplest
  Reset1 : InportShadow  Port=5
  atan2 : mcbcontrolslib/atan2  ApproximationMethod=None  NumberOfIterations=11  NumberOfDataPoints=16  InterpMethod=Flat  outputUnit=PerUnit  TableDataTypeStr=Inherit: Inherit via input
  psiAlpha : Subsystem
  psiBeta : Subsystem
  scaling1 : InportShadow  Port=6
  Position : Outport
  wires:
  scaling/1 -> psiAlpha/4(scaling)
  Ialpha/1 -> psiAlpha/3(Ialpha)
  Ibeta/1 -> psiBeta/2(Ibeta)
  Valpha/1 -> psiAlpha/2(Valpha)
  Reset/1 -> psiBeta/3(Reset)
  Vbeta/1 -> psiBeta/1(Vbeta)
  atan2/1 -> PositionGain/1
  PositionGain/1 -> Position/1
  scaling1/1 -> psiBeta/4(scaling)
  Reset1/1 -> psiAlpha/1(Reset)
  scalingLd/1 -> psiBeta/5(scalingLd), psiAlpha/5(scalingLd)
  psiBeta/1(psiBeta) -> atan2/1
  psiAlpha/1(psiAlpha) -> atan2/2

== system nucleo_g431re_ihm07m1/Alogrithm/Control Algorithm/Flux Observer/FluxObvserver/SpeedMeasurementSubsystem ==
  V_alpha : Inport
  V_beta : Inport  Port=2
  Data Store Read : DataStoreRead  DataStoreName=speed_rated  IndexOptions=Index vector (dialog)  Indices=1  OutputSizes=1
  Data Store Read1 : DataStoreRead  DataStoreName=pole_pairs  IndexOptions=Index vector (dialog)  Indices=1  OutputSizes=1
  Divide : Product  Inputs=*/
  IIR Filter : mcbcontrolslib/IIR Filter  VariantControl=Low Pass Filter  VariantSelect=Low-pass  FilterConstantInputType=Specify via dialog  Filter_constant=0.01*(Ts/(50e-6))  advancedSettings=off  Ts=50e-6  cutOff_freq=64.9612
  Speed_measurement : Subsystem
  atan2 : mcbcontrolslib/atan2  ApproximationMethod=None  NumberOfIterations=11  NumberOfDataPoints=16  InterpMethod=Flat  outputUnit=PerUnit  TableDataTypeStr=Inherit: Inherit via input
  Speed : Outport
  wires:
  Data Store Read1/1 -> Divide/2
  IIR Filter/1 -> Divide/1
  Divide/1 -> Speed/1
  atan2/1 -> Speed_measurement/1(PositionPU)
  V_beta/1 -> atan2/1
  Speed_measurement/1(speedPU) -> IIR Filter/1
  V_alpha/1 -> atan2/2
  Data Store Read/1 -> Speed_measurement/2(MaxSpeed)

== system nucleo_g431re_ihm07m1/Alogrithm/Control Algorithm/Generating Raw Space Vectors/ClarkePark/Pole_Voltage to Phase_Voltage ==
  Vao : Inport
  Vbo : Inport  Port=2
  Vco : Inport  Port=3
  Gain2 : Gain  Gain=1/3  RndMeth=Simplest  OutDataTypeStr=Inherit: Same as input
  Gain3 : Gain  Gain=1/3  RndMeth=Simplest  OutDataTypeStr=Inherit: Same as input
  Sum{,1..4} (5 alike) : Sum  Inputs=|+-
  Va : Outport  VectorParamsAs1DForOutWhenUnconnected=off
  Vb : Outport  Port=2  VectorParamsAs1DForOutWhenUnconnected=off
  wires:
  Sum1/1 -> Sum4/1  "Vbc"
  Sum2/1 -> Sum3/2  "Vca"
  Sum3/1 -> Gain2/1
  Gain3/1 -> Vb/1  "Vb"
  Sum/1 -> Sum3/1, Sum4/2  "Vab"
  Vco/1 -> Sum1/2, Sum2/1
  Sum4/1 -> Gain3/1
  Gain2/1 -> Va/1  "Va"
  Vbo/1 -> Sum/2, Sum1/1
  Vao/1 -> Sum/1, Sum2/2

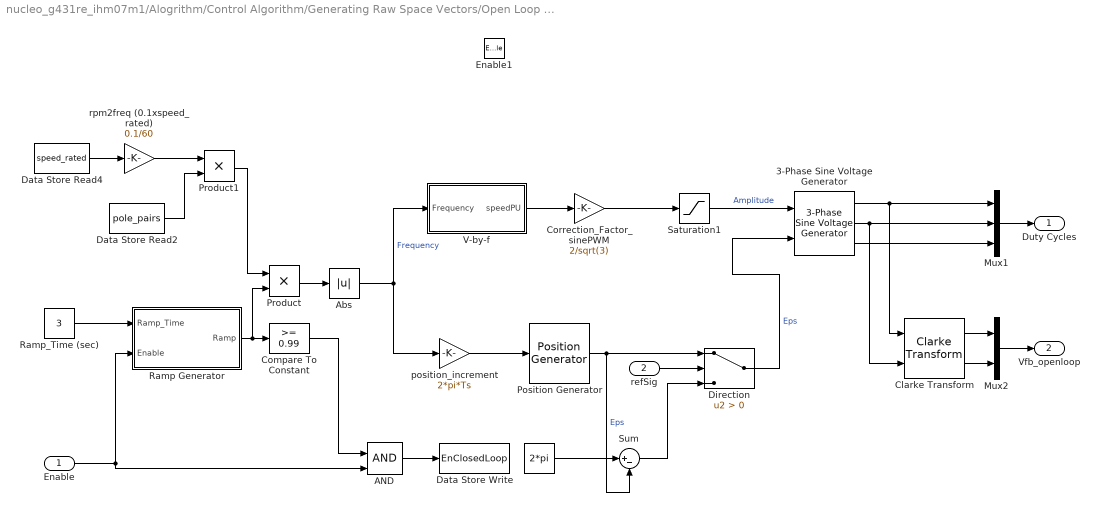
== system nucleo_g431re_ihm07m1/Alogrithm/Control Algorithm/Generating Raw Space Vectors/Open Loop Start-Up/Open Loop Start-Up ==
  Enable : Inport
  refSig : Inport  Port=2
  Enable1 : EnablePort
  " " : Constant  Value=2*pi  OutDataTypeStr=single  SampleTime=-1
  3-Phase Sine Voltage Generator : mcbcontrolslib/3-Phase Sine Voltage Generator  AngleInput=Radians  N_points=1024
  AND : Logic  IconShape=distinctive  AllPortsSameDT=off  OutDataTypeStr=boolean
  Abs : Abs  SaturateOnIntegerOverflow=off
  Clarke Transform : mcbcontrolslib/Clarke Transform  VariantControl=Variant2  PhaseInput=Two inputs  EnPowerInv=off
  Compare To Constant : simulink/Logic and Bit Operations/Compare To Constant  relop=>=  const=0.99  OutDataTypeStr=boolean
  Correction_Factor_sinePWM : Gain  Gain=2/sqrt(3)  ParamDataTypeStr=single  RndMeth=Simplest  OutDataTypeStr=Inherit: Same as input
  Data Store Read2 : DataStoreRead  DataStoreName=pole_pairs  IndexOptions=Index vector (dialog)  Indices=1  OutputSizes=1
  Data Store Read4 : DataStoreRead  DataStoreName=speed_rated  IndexOptions=Index vector (dialog)  Indices=1  OutputSizes=1
  Data Store Write : DataStoreWrite  DataStoreName=EnClosedLoop  IndexOptions=Index vector (dialog)  Indices=1  OutputSizes=1
  Direction : Switch  Criteria=u2 > Threshold  OutDataTypeStr=single  RndMeth=Simplest  SaturateOnIntegerOverflow=off  InputSameDT=off
  Mux1 : Mux  Inputs=3
  Mux2 : Mux  Inputs=2
  Position Generator : mcbcontrolslib/Position Generator  AngleOutput=Radians  ExternalReset=none  Offset=0
  Product : Product  RndMeth=Simplest  OutDataTypeStr=Inherit: Same as first input
  Product1 : Product  RndMeth=Simplest  OutDataTypeStr=Inherit: Same as first input
  Ramp Generator : Subsystem
  Ramp_Time (sec) : Constant  Value=3  OutDataTypeStr=single  SampleTime=-1
  Saturation1 : Saturate  UpperLimit=0.95  LowerLimit=0.1  RndMeth=Simplest
  Sum : Sum  Inputs=|+-  RndMeth=Simplest  OutDataTypeStr=Inherit: Same as first input
  V-by-f : Subsystem
  position_increment : Gain  Gain=2*pi*Ts  RndMeth=Simplest  OutDataTypeStr=Inherit: Same as input
  rpm2freq (0.1xspeed_rated) : Gain  Gain=0.1/60  RndMeth=Simplest  OutDataTypeStr=Inherit: Same as input
  Duty Cycles : Outport  VectorParamsAs1DForOutWhenUnconnected=off
  Vfb_openloop : Outport  Port=2  VectorParamsAs1DForOutWhenUnconnected=off
  wires:
  3-Phase Sine Voltage Generator/1 -> Clarke Transform/1, Mux1/1
  3-Phase Sine Voltage Generator/3 -> Mux1/3
  Direction/1 -> 3-Phase Sine Voltage Generator/2  "Eps"
  Saturation1/1 -> 3-Phase Sine Voltage Generator/1  "Amplitude"
  Mux1/1 -> Duty Cycles/1
  Ramp Generator/1(Ramp) -> Compare To Constant/1, Product/2
  Ramp_Time (sec)/1 -> Ramp Generator/1(Ramp_Time)
  Position Generator/1 -> Sum/2, Direction/1  "Eps"
  " "/1 -> Sum/1
  Sum/1 -> Direction/3
  Abs/1 -> V-by-f/1(Frequency), position_increment/1  "Frequency"
  position_increment/1 -> Position Generator/1
  Product/1 -> Abs/1
  Product1/1 -> Product/1
  refSig/1 -> Direction/2
  Compare To Constant/1 -> AND/1
  3-Phase Sine Voltage Generator/2 -> Clarke Transform/2, Mux1/2
  Clarke Transform/1 -> Mux2/1
  Clarke Transform/2 -> Mux2/2
  Mux2/1 -> Vfb_openloop/1
  Data Store Read4/1 -> rpm2freq (0.1xspeed_rated)/1
  rpm2freq (0.1xspeed_rated)/1 -> Product1/1
  Data Store Read2/1 -> Product1/2
  V-by-f/1(speedPU) -> Correction_Factor_sinePWM/1
  Correction_Factor_sinePWM/1 -> Saturation1/1
  AND/1 -> Data Store Write/1
  Enable/1 -> Ramp Generator/2(Enable), AND/2
